simulink model "Master_Slave_Model"  (R2020b)
settings: Solver=VariableStepAuto  StartTime=0.0  StopTime=10  RelTol=1e-3
values from neighbouring files (symbols this model uses):
  A = [1 Ts;0 1]    [parameters_ACZC.m]
  Be = 5    [parameters_ACZC.m]
  beta = 2*pi*Fc*Ts / (1+2*pi*Fc*Ts)    (= 0.111635211705)    [parameters_ACZC.m]
  Bh = 2*0.7*sqrt(Kh)    [parameters_ACZC.m]
  C = [1 0]    [parameters_ACZC.m]
  delayCommM2S = 0    [parameters_ACZC.m]
  delayCommS2M = 0    [parameters_ACZC.m]
  dt = 0.001    [parameters_ACZC.m]
  Fc = 20    [parameters_ACZC.m]
  Jh = 0    [parameters_ACZC.m]
  k_m = 19.34    [parameters_ACZC.m]
  k_s = 19.34    [parameters_ACZC.m]
  Kc2v_m = 2    [parameters_ACZC.m]
  Kc2v_s = 2    [parameters_ACZC.m]
  Kd_h = 0.5    [parameters_ACZC.m]
  Kd_s = 1.5    [parameters_ACZC.m]
  Ke = 10    [parameters_ACZC.m]
  Kh = 2    [parameters_ACZC.m]
  Kh_max = 50    [parameters_ACZC.m]
  Kp_h = 1.2    [parameters_ACZC.m]
  Kp_s = 1    [parameters_ACZC.m]
  Kt2c_m = 1.182    [parameters_ACZC.m]
  Kt2c_s = 1.182    [parameters_ACZC.m]
  lArm_m = 0.1    [parameters_ACZC.m]
  lArm_s = 0.1    [parameters_ACZC.m]
  maxCurrent_m = 4.5    [parameters_ACZC.m]
  maxCurrent_s = 4.5    [parameters_ACZC.m]
  PosRef = 1    [parameters_ACZC.m]
  qe = 2    [parameters_ACZC.m]
  stopTime = str2double(stopTime)    [parameters_ACZC.m]
  tau_s = 1.217    [parameters_ACZC.m]
  Ts = 0.001    [parameters_ACZC.m]
  Variance = 0.0000001    (= 1e-07)    [parameters_ACZC.m]
undefined symbols (not defined in the file or in its folder): DiscIntNeverNeededParam, Discrete, Time
libraries: simulink_extras x20, dspsigops x20, ctrlSharedLib x7, cstblocks x1
settings Model: Creator=Mirko  LastModifiedBy=mirko

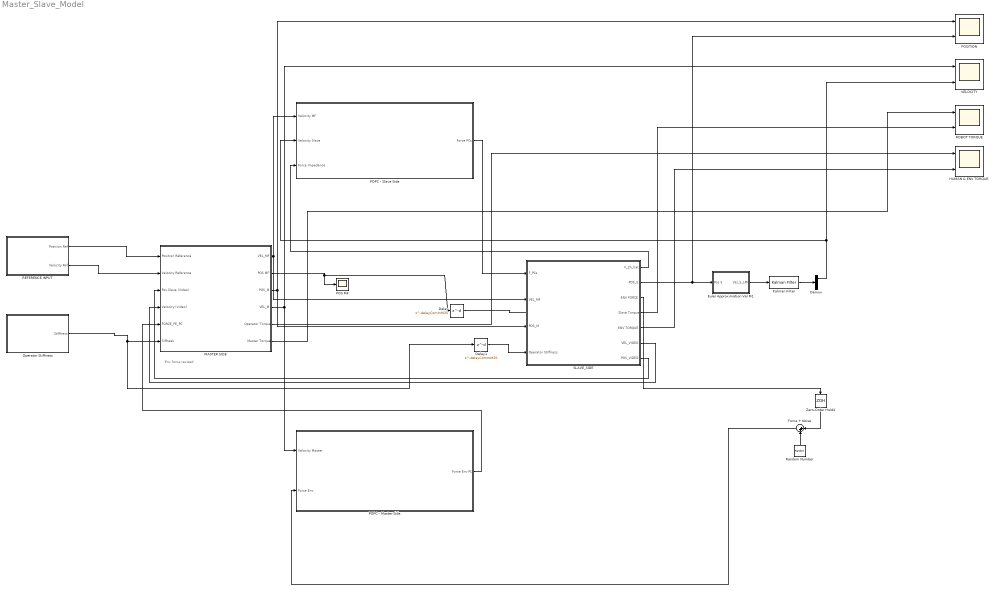
== system Master_Slave_Model ==
  note: Env force revised
  Delay : Delay  DelayLength=delayCommM2S  SampleTime=Ts
  Delay1 : Delay  DelayLength=delayCommM2S  SampleTime=Ts
  Demux : Demux  Outputs=2
  Euler Approximation Vel M1 : Subsystem
  Force + Noise : Sum  Inputs=|++
  HUMAN & ENV TORQUE : Scope  NumInputPorts=2
  Kalman Filter : ctrlSharedLib/Kalman Filter  TimeDomain=Discrete-Time  UseCurrentEstimator=off  ModelSource=Individual A, B, C, D matrices  ModelSourceVariable=ss(A,0,C,0)  A=A  B=1  C=C  D=0  NumberOfStates=2  NumberOfInputs=1  NumberOfOutputs=1  InitialEstimateSource=Dialog  X0=0  P0=10  UseK=off  UseGH=off  NumberOfProcessNoiseInputs=1  G=1  TimeInvariantG=on  H=0  TimeInvariantH=on  Q=0.05  TimeInvariantQ=on  R=1  TimeInvariantR=on  N=0  TimeInvariantN=on  AddInputPort=off  AddEnablePort=off  OutputEstimatedY=off  OutputP=off  Ts=Ts
  MASTER SIDE : Subsystem
  Operator Stiffness : Subsystem
  POPC - Master Side : Subsystem
  POPC - Slave Side : Subsystem
  "POS MF " : Scope
  "POSITION " : Scope  NumInputPorts=2
  REFERENCE INPUT : Subsystem
  ROBOT TORQUE : Scope  NumInputPorts=2
  Random Number : RandomNumber  Variance=Variance  SampleTime=Ts
  "SLAVE_SIDE " : Subsystem
  VELOCITY : Scope  NumInputPorts=2
  Zero-Order Hold4 : ZeroOrderHold  SampleTime=Ts
  wires:
  Delay1/1 -> "SLAVE_SIDE "/4(Operator Stiffness)
  Delay/1 -> ?
  Operator Stiffness/1(Stiffness) -> Delay1/1, MASTER SIDE/6(Siffness)
  "SLAVE_SIDE "/1(F_Zh_hat) -> POPC - Slave Side/3(Force Impedence)
  MASTER SIDE/2(POS MF) -> "POS MF "/1, Delay/1
  "SLAVE_SIDE "/2(POS_S) -> "POSITION "/2, Euler Approximation Vel M1/1(Pos S)
  MASTER SIDE/1(VEL_MF) -> "SLAVE_SIDE "/2(VEL_MF), POPC - Slave Side/1(Velocity MF)
  Demux/1 -> VELOCITY/2, POPC - Slave Side/2(Velocity Slave)
  Kalman Filter/1 -> Demux/1
  Euler Approximation Vel M1/1("Vel_S_LPF ") -> Kalman Filter/1
  POPC - Slave Side/1(Force PCs) -> "SLAVE_SIDE "/1(F_PCs)
  MASTER SIDE/4(VEL_M) -> POPC - Master Side/1(Velocity Master), VELOCITY/1
  Force + Noise/1 -> POPC - Master Side/2(Force Env)
  Zero-Order Hold4/1 -> Force + Noise/1
  Random Number/1 -> Force + Noise/2
  "SLAVE_SIDE "/3(ENV FORCE) -> Zero-Order Hold4/1
  POPC - Master Side/1(Force Env PC) -> MASTER SIDE/5("FORCE_FE_PC ")
  MASTER SIDE/3(POS_M) -> "SLAVE_SIDE "/3(POS_M), "POSITION "/1
  MASTER SIDE/5(Operator Torque) -> HUMAN & ENV TORQUE/1
  MASTER SIDE/6(Master Torque) -> ROBOT TORQUE/1
  REFERENCE INPUT/1("Position Ref ") -> MASTER SIDE/1(Position Reference)
  REFERENCE INPUT/2("Velocity Ref ") -> MASTER SIDE/2(Velocity Reference)
  "SLAVE_SIDE "/7(POS_VIDEO) -> MASTER SIDE/3(Pos Slave (Video))
  "SLAVE_SIDE "/6(VEL_VIDEO) -> MASTER SIDE/4(Velocity (Video))
  "SLAVE_SIDE "/4(Slave Torque) -> ROBOT TORQUE/2
  "SLAVE_SIDE "/5(ENV TORQUE) -> HUMAN & ENV TORQUE/2

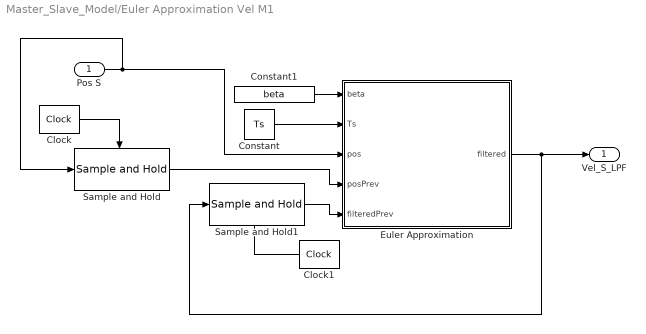
== system Master_Slave_Model/Euler Approximation Vel M1 ==
  Pos S : Inport
  Clock : simulink_extras/Flip Flops/Clock  period=Ts*2
  Clock1 : simulink_extras/Flip Flops/Clock  period=Ts*2
  Constant : Constant  Value=Ts
  Constant1 : Constant  Value=beta
  "Euler Approximation " : MATLAB Function  TreatAsAtomicUnit=on
  Sample and Hold : dspsigops/Sample and Hold  trig=Rising edge  initCond=0  latchinput=on
  Sample and Hold1 : dspsigops/Sample and Hold  trig=Rising edge  initCond=0  latchinput=on
  "Vel_S_LPF " : Outport
  wires:
  Pos S/1 -> Sample and Hold/1, "Euler Approximation "/3(pos)
  Constant/1 -> "Euler Approximation "/2(Ts)
  Sample and Hold/1 -> "Euler Approximation "/4(posPrev)
  Clock/1 -> Sample and Hold/Trigger
  Sample and Hold1/1 -> "Euler Approximation "/5(filteredPrev)
  "Euler Approximation "/1(filtered) -> "Vel_S_LPF "/1, Sample and Hold1/1
  Clock1/1 -> Sample and Hold1/Trigger
  Constant1/1 -> "Euler Approximation "/1(beta)

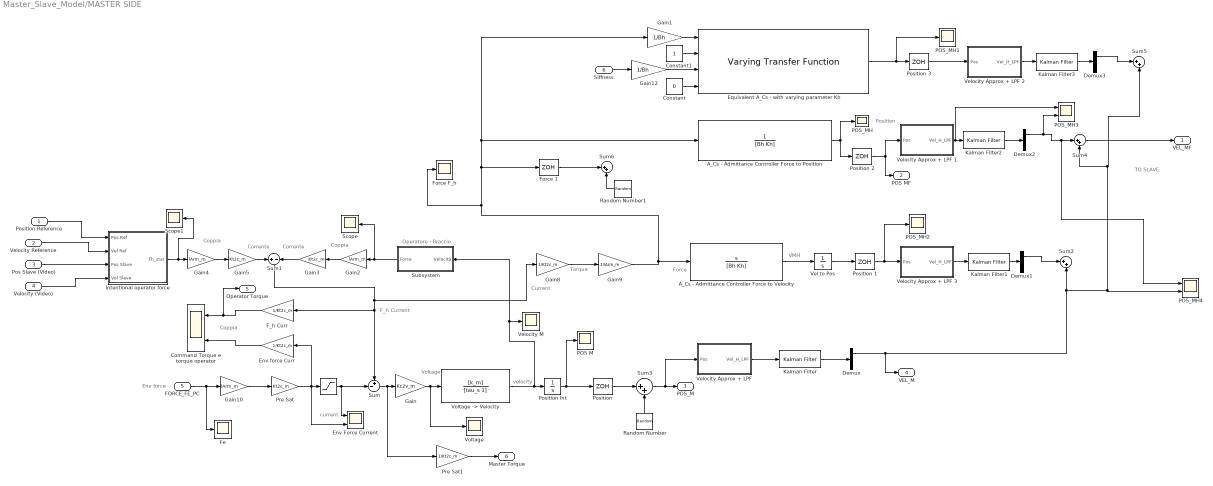
== system Master_Slave_Model/MASTER SIDE ==
  note: VMH
  note: Position
  note: Env force
  note: Force
  note: Torque
  note: Current
  note: F_h Current
  note: Coppia
  note: Corrente
  note: Coppia
  note: Corrente
  note: Coppia
  note: Operatore - Braccio
  note: current
  note: Voltage
  note: velocity
  note: TO SLAVE
  Position Reference : Inport
  Velocity Reference : Inport  Port=2
  Pos Slave (Video) : Inport  Port=3
  Velocity (Video) : Inport  Port=4
  "FORCE_FE_PC " : Inport  Port=5
  Siffness : Inport  Port=6
  " " : Saturate  UpperLimit=maxCurrent_m  LowerLimit=-maxCurrent_m
  A_Cs - Admittance Controller Force to Position : TransferFcn  Denominator=[Bh Kh]
  A_Cs - Admittance Controller Force to Velocity : TransferFcn  Numerator=[1 0]  Denominator=[Bh Kh]
  "Command Torque e torque operator " : Scope  NumInputPorts=2
  Constant : Constant  Value=0
  Constant1 : Constant
  Demux{,1..3} (4 alike) : Demux  Outputs=2
  Env Force Current : Scope  NumInputPorts=2
  Env force Curr : Gain  Gain=1/Kt2c_m
  Equivalent A_Cs - with varying parameter Kh : cstblocks/Linear Parameter Varying/Varying Transfer Function  N=1
  F_h Curr : Gain  Gain=1/Kt2c_m
  Fe : Scope
  Force 1 : ZeroOrderHold  SampleTime=Ts
  "Force F_h " : Scope
  Gain : Gain  Gain=Kc2v_m
  Gain1 : Gain  Gain=1/Bh
  Gain10 : Gain  Gain=lArm_m
  Gain12 : Gain  Gain=1/Bh
  Gain2 : Gain  Gain=lArm_m
  Gain3 : Gain  Gain=Kt2c_m
  Gain4 : Gain  Gain=lArm_m
  Gain5 : Gain  Gain=Kt2c_m
  Gain8 : Gain  Gain=1/Kt2c_m
  Gain9 : Gain  Gain=1/lArm_m
  Intentional operator force : Subsystem
  Kalman Filter{,1..3} (4 alike) : ctrlSharedLib/Kalman Filter  TimeDomain=Discrete-Time  UseCurrentEstimator=off  ModelSource=Individual A, B, C, D matrices  ModelSourceVariable=ss(A,0,C,0)  A=A  B=1  C=C  D=0  NumberOfStates=2  NumberOfInputs=1  NumberOfOutputs=1  InitialEstimateSource=Dialog  X0=0  P0=10  UseK=off  UseGH=off  NumberOfProcessNoiseInputs=1  G=1  TimeInvariantG=on  H=0  TimeInvariantH=on  Q=0.05  TimeInvariantQ=on  R=1  TimeInvariantR=on  N=0  TimeInvariantN=on  AddInputPort=off  AddEnablePort=off  OutputEstimatedY=off  OutputP=off  Ts=Ts
  "POS M " : Scope
  POS_MH : Scope
  POS_MH1 : Scope
  POS_MH2 : Scope
  POS_MH3 : Scope  NumInputPorts=2
  POS_MH4 : Scope  NumInputPorts=2
  Position {,1..3} (4 alike) : ZeroOrderHold  SampleTime=Ts
  "Position Int " : Integrator
  Pre Sat : Gain  Gain=Kt2c_m
  Pre Sat1 : Gain  Gain=1/Kt2c_m
  Random Number : RandomNumber  Variance=Variance  SampleTime=Ts
  Random Number1 : RandomNumber  Variance=Variance  SampleTime=0.1
  Scope : Scope
  Scope1 : Scope
  Subsystem : Subsystem
  Sum : Sum  Inputs=+-|
  Sum1 : Sum  Inputs=+-
  Sum{2..6} (5 alike) : Sum  Inputs=|++
  Vel to Pos : Integrator
  "Velocity Approx + LPF " : Subsystem
  Velocity Approx + LPF 1 : Subsystem
  Velocity Approx + LPF 2 : Subsystem
  Velocity Approx + LPF 3 : Subsystem
  Velocity M : Scope
  Voltage : Scope
  "Voltage -> Velocity" : TransferFcn  Numerator=[k_m]  Denominator=[tau_s 1]
  VEL_MF : Outport
  POS MF : Outport  Port=2
  POS_M : Outport  Port=3
  VEL_M : Outport  Port=4
  Operator Torque : Outport  Port=5
  Master Torque : Outport  Port=6
  wires:
  Pre Sat/1 -> Env Force Current/2, Env force Curr/1, " "/1
  "Position Int "/1 -> "Position "/1, "POS M "/1
  "Voltage -> Velocity"/1 -> Velocity M/1, Subsystem/1("Velocità "), "Position Int "/1
  Sum1/1 -> Sum/1, F_h Curr/1, Gain8/1
  Gain4/1 -> Gain5/1
  F_h Curr/1 -> Operator Torque/1, "Command Torque e torque operator "/1
  Gain2/1 -> Gain3/1
  Gain3/1 -> Sum1/2
  Env force Curr/1 -> "Command Torque e torque operator "/2
  Gain5/1 -> Sum1/1
  Gain/1 -> "Voltage -> Velocity"/1, Voltage/1
  Velocity Approx + LPF 3/1("Vel_H_LPF ") -> Kalman Filter1/1
  Gain8/1 -> Gain9/1
  Gain9/1 -> Force 1/1, Gain1/1, A_Cs - Admittance Controller Force to Position/1, "Force F_h "/1, A_Cs - Admittance Controller Force to Velocity/1
  "FORCE_FE_PC "/1 -> Fe/1, Gain10/1
  Gain10/1 -> Pre Sat/1
  Constant/1 -> Equivalent A_Cs - with varying parameter Kh/4
  Gain12/1 -> Equivalent A_Cs - with varying parameter Kh/3
  Siffness/1 -> Gain12/1
  Constant1/1 -> Equivalent A_Cs - with varying parameter Kh/2
  Equivalent A_Cs - with varying parameter Kh/1 -> Position 3/1, POS_MH1/1
  Subsystem/1(Force) -> Scope/1, Gain2/1
  A_Cs - Admittance Controller Force to Position/1 -> Position 2/1, POS_MH/1
  Sum4/1 -> VEL_MF/1
  Gain1/1 -> Equivalent A_Cs - with varying parameter Kh/1
  Velocity Approx + LPF 1/1("Vel_H_LPF ") -> POS_MH3/1, Kalman Filter2/1
  Velocity Approx + LPF 2/1("Vel_H_LPF ") -> Kalman Filter3/1
  " "/1 -> Sum/2, Env Force Current/1
  Random Number/1 -> Sum3/2
  Sum3/1 -> "Velocity Approx + LPF "/1(Pos), POS_M/1
  "Velocity Approx + LPF "/1("Vel_H_LPF ") -> Kalman Filter/1
  "Position "/1 -> Sum3/1
  Velocity (Video)/1 -> Intentional operator force/4(Vel Slave)
  Pos Slave (Video)/1 -> Intentional operator force/3(Pos Slave)
  Position Reference/1 -> Intentional operator force/1(Pos Ref)
  Velocity Reference/1 -> Intentional operator force/2(Vel Ref)
  Intentional operator force/1("Fh_star ") -> Scope1/1, Gain4/1
  Random Number1/1 -> Sum6/2
  Force 1/1 -> Sum6/1
  Demux/1 -> Sum2/2, Sum4/2, Sum5/2, POS_MH4/2, VEL_M/1
  Kalman Filter/1 -> Demux/1
  A_Cs - Admittance Controller Force to Velocity/1 -> Vel to Pos/1
  Position 1/1 -> Velocity Approx + LPF 3/1(Pos), POS_MH2/1
  Demux1/1 -> Sum2/1
  Kalman Filter1/1 -> Demux1/1
  Demux2/1 -> POS_MH3/2, POS_MH4/1, Sum4/1
  Kalman Filter2/1 -> Demux2/1
  Vel to Pos/1 -> Position 1/1
  Position 2/1 -> Velocity Approx + LPF 1/1(Pos), POS MF/1
  Position 3/1 -> Velocity Approx + LPF 2/1(Pos)
  Demux3/1 -> Sum5/1
  Kalman Filter3/1 -> Demux3/1
  Pre Sat1/1 -> Master Torque/1
  Sum/1 -> Pre Sat1/1, Gain/1

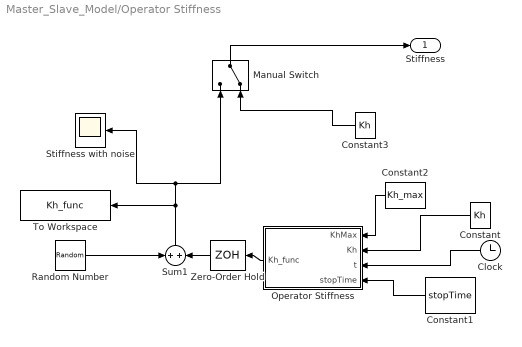
== system Master_Slave_Model/Operator Stiffness ==
  Clock : Clock
  Constant : Constant  Value=Kh
  Constant1 : Constant  Value=stopTime  SampleTime=Ts
  Constant2 : Constant  Value=Kh_max
  Constant3 : Constant  Value=Kh
  Manual Switch : ManualSwitch  CurrentSetting=0
  "Operator Stiffness " : MATLAB Function  TreatAsAtomicUnit=on
  Random Number : RandomNumber  Variance=Variance  SampleTime=Ts
  Stiffness with noise : Scope
  Sum1 : Sum
  To Workspace : ToWorkspace  VariableName=Kh_func  SaveFormat=Structure With Time  SampleTime=-1
      settings: Save2DSignal=2-D array (concatenate along first dimension)
  Zero-Order Hold : ZeroOrderHold  SampleTime=-1
  Stiffness : Outport
  wires:
  Constant3/1 -> Manual Switch/2
  Sum1/1 -> To Workspace/1, Manual Switch/1, Stiffness with noise/1
  Constant2/1 -> "Operator Stiffness "/1(KhMax)
  "Operator Stiffness "/1(Kh_func) -> Zero-Order Hold/1
  Clock/1 -> "Operator Stiffness "/3(t)
  Random Number/1 -> Sum1/1
  Constant/1 -> "Operator Stiffness "/2(Kh)
  Constant1/1 -> "Operator Stiffness "/4(stopTime)
  Manual Switch/1 -> Stiffness/1
  Zero-Order Hold/1 -> Sum1/2

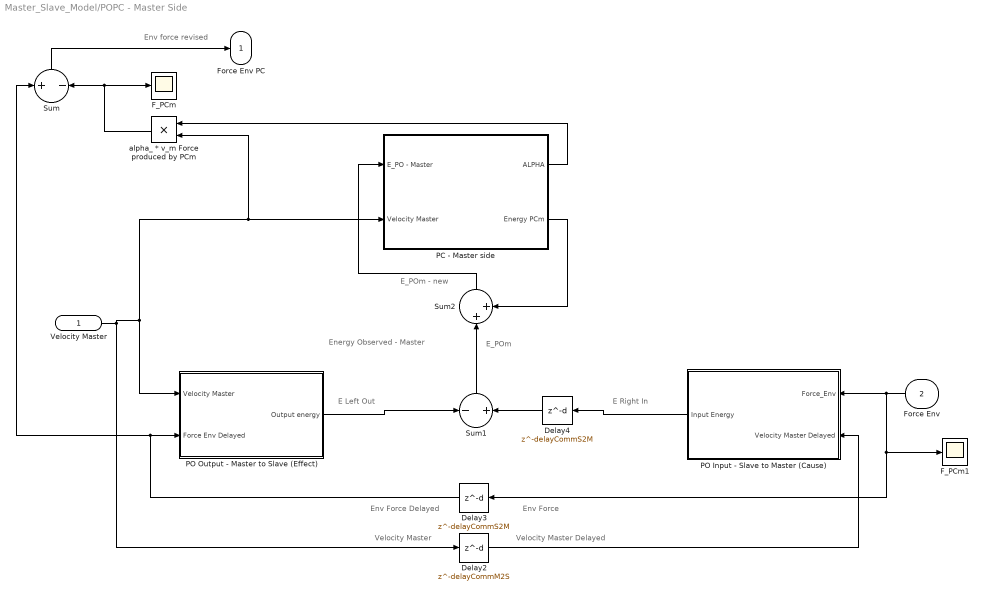
== system Master_Slave_Model/POPC - Master Side ==
  note: E_POm
  note: Energy Observed - Master
  note: Env force revised
  note: Env Force Delayed
  note: Env Force
  note: Velocity Master
  note: Velocity Master Delayed
  note: E Left Out
  note: E Right In
  note: E_POm - new
  Velocity Master : Inport
  Force Env : Inport  Port=2
  Delay2 : Delay  DelayLength=delayCommM2S  InitialCondition=0  SampleTime=Ts
  Delay3 : Delay  DelayLength=delayCommS2M  InitialCondition=0  SampleTime=Ts
  Delay4 : Delay  DelayLength=delayCommS2M  InitialCondition=0
  F_PCm : Scope
  F_PCm1 : Scope
  PC - Master side : Subsystem
  PO Input - Slave to Master (Cause) : Subsystem
  PO Output - Master to Slave (Effect) : Subsystem
  Sum : Sum  Inputs=+-
  Sum1 : Sum  Inputs=-+
  Sum2 : Sum  Inputs=|++
  alpha_ * v_m Force produced by PCm : Product
  Force Env PC : Outport
  wires:
  alpha_ * v_m Force produced by PCm/1 -> Sum/2, F_PCm/1
  Force Env/1 -> Delay3/1, F_PCm1/1, PO Input - Slave to Master (Cause)/1(Force_Env)
  Delay3/1 -> Sum/1, PO Output - Master to Slave (Effect)/2(Force Env Delayed)
  Velocity Master/1 -> Delay2/1, alpha_ * v_m Force produced by PCm/2, PC - Master side/2("Velocity Master "), PO Output - Master to Slave (Effect)/1(Velocity Master)
  Sum1/1 -> Sum2/1
  Sum/1 -> Force Env PC/1
  PO Output - Master to Slave (Effect)/1(Output energy) -> Sum1/1
  Delay4/1 -> Sum1/2
  Delay2/1 -> PO Input - Slave to Master (Cause)/2(Velocity Master Delayed)
  PO Input - Slave to Master (Cause)/1(Input Energy) -> Delay4/1
  Sum2/1 -> PC - Master side/1(E_PO - Master)
  PC - Master side/1(ALPHA) -> alpha_ * v_m Force produced by PCm/1
  PC - Master side/2(Energy PCm) -> Sum2/2

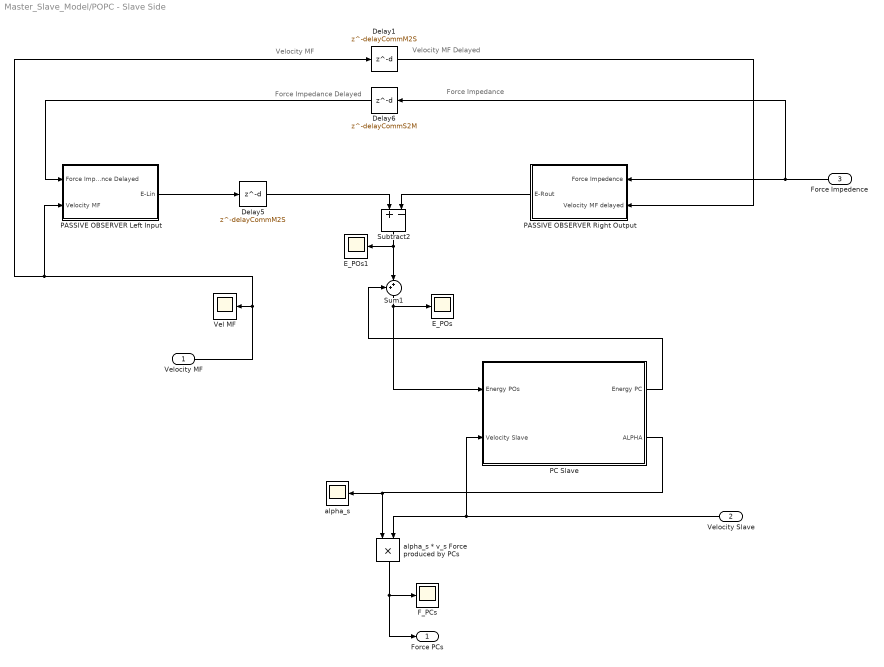
== system Master_Slave_Model/POPC - Slave Side ==
  note: Velocity MF Delayed
  note: Velocity MF
  note: Force Impedance Delayed
  note: Force Impedance
  Velocity MF : Inport
  Velocity Slave : Inport  Port=2
  Force Impedence : Inport  Port=3
  Delay1 : Delay  DelayLength=delayCommM2S  InitialCondition=0  SampleTime=Ts
  Delay5 : Delay  DelayLength=delayCommM2S  InitialCondition=0  SampleTime=Ts
  Delay6 : Delay  DelayLength=delayCommS2M  InitialCondition=0  SampleTime=Ts
  E_POs : Scope
  E_POs1 : Scope
  F_PCs : Scope
  PASSIVE OBSERVER Left Input : Subsystem
  PASSIVE OBSERVER Right Output : Subsystem
  PC Slave : Subsystem
  Subtract2 : Sum  Inputs=+|-
  Sum1 : Sum  Inputs=++|
  Vel MF : Scope
  alpha_s : Scope
  alpha_s * v_s Force produced by PCs : Product
  Force PCs : Outport
  wires:
  Subtract2/1 -> E_POs1/1, Sum1/2
  Delay6/1 -> PASSIVE OBSERVER Left Input/1(Force Impedance Delayed)
  Velocity Slave/1 -> alpha_s * v_s Force produced by PCs/2, PC Slave/2(Velocity Slave)
  Sum1/1 -> PC Slave/1(Energy POs), E_POs/1
  Delay5/1 -> Subtract2/1
  alpha_s * v_s Force produced by PCs/1 -> Force PCs/1, F_PCs/1
  PASSIVE OBSERVER Left Input/1(E-Lin) -> Delay5/1
  Velocity MF/1 -> PASSIVE OBSERVER Left Input/2(Velocity MF), Delay1/1, Vel MF/1
  PASSIVE OBSERVER Right Output/1(E-Rout) -> Subtract2/2
  Force Impedence/1 -> Delay6/1, PASSIVE OBSERVER Right Output/1(Force Impedence)
  Delay1/1 -> PASSIVE OBSERVER Right Output/2(Velocity MF delayed)
  PC Slave/2(ALPHA) -> alpha_s * v_s Force produced by PCs/1, alpha_s/1
  PC Slave/1(Energy PC) -> Sum1/1

== system Master_Slave_Model/REFERENCE INPUT ==
  Derivative : Derivative
  Manual Switch : ManualSwitch  CurrentSetting=0
  Scope : Scope
  Sine Wave : Sin  Amplitude=PosRef  SampleTime=0
  Step : Step  After=PosRef  SampleTime=0
  Transfer Fcn : TransferFcn  Numerator=[2*pi*Fc]  Denominator=[1 2*pi*Fc]
  "Position Ref " : Outport
  "Velocity Ref " : Outport  Port=2
  wires:
  Sine Wave/1 -> Manual Switch/1
  Derivative/1 -> "Velocity Ref "/1
  Manual Switch/1 -> Derivative/1, "Position Ref "/1
  Transfer Fcn/1 -> Scope/1, Manual Switch/2
  Step/1 -> Transfer Fcn/1

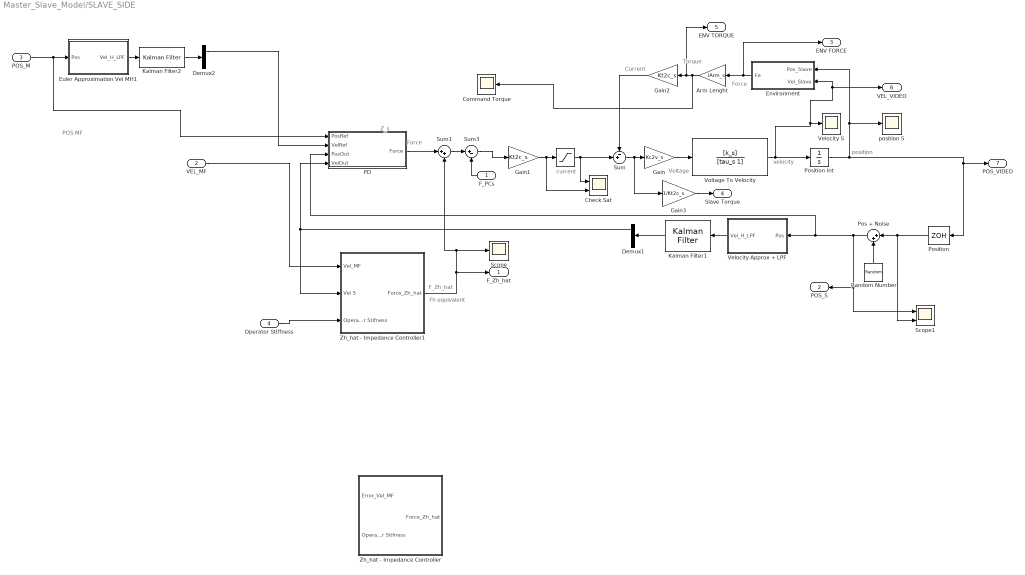
== system Master_Slave_Model/SLAVE_SIDE  ==
  note: Fh equivalent
  note: POS MF
  note: current
  note: Force
  note: velocity
  note: position
  note: Current
  note: Voltage
  note: Torque
  note: Z_s
  note: Force
  note: F_Zh_hat
  F_PCs : Inport
  VEL_MF : Inport  Port=2
  POS_M : Inport  Port=3
  Operator Stiffness : Inport  Port=4
  " " : Saturate  UpperLimit=maxCurrent_s  LowerLimit=-maxCurrent_s
  Arm Lenght : Gain  Gain=lArm_s
  Check Sat : Scope  NumInputPorts=2
  Command Torque : Scope
  Demux1 : Demux  Outputs=2
  Demux2 : Demux  Outputs=2
  "Environment " : Subsystem
  Euler Approximation Vel MH1 : Subsystem
  Gain : Gain  Gain=Kc2v_s
  Gain1 : Gain  Gain=Kt2c_s
  Gain2 : Gain  Gain=Kt2c_s
  Gain3 : Gain  Gain=1/Kt2c_s
  Kalman Filter1 : ctrlSharedLib/Kalman Filter  TimeDomain=Discrete-Time  UseCurrentEstimator=off  ModelSource=Individual A, B, C, D matrices  ModelSourceVariable=ss(A,0,C,0)  A=A  B=1  C=C  D=0  NumberOfStates=2  NumberOfInputs=1  NumberOfOutputs=1  InitialEstimateSource=Dialog  X0=0  P0=10  UseK=off  UseGH=off  NumberOfProcessNoiseInputs=1  G=1  TimeInvariantG=on  H=0  TimeInvariantH=on  Q=0.05  TimeInvariantQ=on  R=1  TimeInvariantR=on  N=0  TimeInvariantN=on  AddInputPort=off  AddEnablePort=off  OutputEstimatedY=off  OutputP=off  Ts=Ts
  Kalman Filter2 : ctrlSharedLib/Kalman Filter  TimeDomain=Discrete-Time  UseCurrentEstimator=off  ModelSource=Individual A, B, C, D matrices  ModelSourceVariable=ss(A,0,C,0)  A=A  B=1  C=C  D=0  NumberOfStates=2  NumberOfInputs=1  NumberOfOutputs=1  InitialEstimateSource=Dialog  X0=0  P0=10  UseK=off  UseGH=off  NumberOfProcessNoiseInputs=1  G=1  TimeInvariantG=on  H=0  TimeInvariantH=on  Q=0.05  TimeInvariantQ=on  R=1  TimeInvariantR=on  N=0  TimeInvariantN=on  AddInputPort=off  AddEnablePort=off  OutputEstimatedY=off  OutputP=off  Ts=Ts
  PD : Subsystem
  Pos + Noise : Sum  Inputs=|++
  Position : ZeroOrderHold  SampleTime=Ts
  "Position Int " : Integrator
  Random Number : RandomNumber  Variance=Variance  SampleTime=Ts
  Scope : Scope
  Scope1 : Scope  NumInputPorts=2
  Sum : Sum  Inputs=-+|
  Sum1 : Sum  Inputs=|++
  Sum3 : Sum  Inputs=|+-
  "Velocity Approx + LPF " : Subsystem
  Velocity S : Scope
  "Voltage To Velocity " : TransferFcn  Numerator=[k_s]  Denominator=[tau_s 1]
  Zh_hat - Impedance Controller : Subsystem
  Zh_hat - Impedance Controller1 : Subsystem
  "position S " : Scope
  F_Zh_hat : Outport
  POS_S : Outport  Port=2
  ENV FORCE : Outport  Port=3
  Slave Torque : Outport  Port=4
  ENV TORQUE : Outport  Port=5
  VEL_VIDEO : Outport  Port=6
  POS_VIDEO : Outport  Port=7
  wires:
  PD/1(Force) -> Sum1/1
  "Position Int "/1 -> Position/1, POS_VIDEO/1, "position S "/1, "Environment "/1(Pos_Slave)
  Gain1/1 -> Check Sat/2, " "/1
  Gain2/1 -> Sum/1
  "Environment "/1(Fe) -> ENV FORCE/1, Arm Lenght/1
  "Voltage To Velocity "/1 -> "Position Int "/1, Velocity S/1, "Environment "/2("Vel_Slave "), VEL_VIDEO/1
  Sum/1 -> Gain3/1, Gain/1
  Gain/1 -> "Voltage To Velocity "/1
  Sum1/1 -> Sum3/1
  " "/1 -> Check Sat/1, Sum/2
  Arm Lenght/1 -> Command Torque/1, ENV TORQUE/1, Gain2/1
  Zh_hat - Impedance Controller1/1("Force_Zh_hat ") -> Sum1/2, Scope/1, F_Zh_hat/1
  F_PCs/1 -> Sum3/2
  Operator Stiffness/1 -> Zh_hat - Impedance Controller1/3(Operator Stifness)
  VEL_MF/1 -> Zh_hat - Impedance Controller1/1(Vel_MF)
  Pos + Noise/1 -> PD/3(PosOut), "Velocity Approx + LPF "/1(Pos), POS_S/1, Scope1/1
  Random Number/1 -> Pos + Noise/2
  Demux1/1 -> PD/4(VelOut), Zh_hat - Impedance Controller1/2(Vel S)
  Position/1 -> Scope1/2, Pos + Noise/1
  "Velocity Approx + LPF "/1("Vel_H_LPF ") -> Kalman Filter1/1
  Kalman Filter1/1 -> Demux1/1
  Gain3/1 -> Slave Torque/1
  POS_M/1 -> PD/1(PosRef), Euler Approximation Vel MH1/1(Pos)
  Euler Approximation Vel MH1/1("Vel_H_LPF ") -> Kalman Filter2/1
  Kalman Filter2/1 -> Demux2/1
  Demux2/1 -> PD/2(VelRef)
  Sum3/1 -> Gain1/1

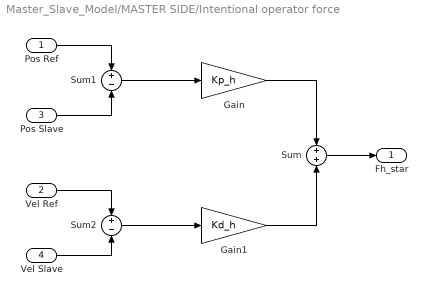
== system Master_Slave_Model/MASTER SIDE/Intentional operator force ==
  Pos Ref : Inport
  Vel Ref : Inport  Port=2
  Pos Slave : Inport  Port=3
  Vel Slave : Inport  Port=4
  Gain : Gain  Gain=Kp_h
  Gain1 : Gain  Gain=Kd_h
  Sum : Sum
  Sum1 : Sum  Inputs=+-
  Sum2 : Sum  Inputs=+-
  "Fh_star " : Outport
  wires:
  Sum/1 -> "Fh_star "/1
  Pos Ref/1 -> Sum1/1
  Pos Slave/1 -> Sum1/2
  Vel Ref/1 -> Sum2/1
  Vel Slave/1 -> Sum2/2
  Sum1/1 -> Gain/1
  Sum2/1 -> Gain1/1
  Gain1/1 -> Sum/2
  Gain/1 -> Sum/1

== system Master_Slave_Model/MASTER SIDE/Subsystem ==
  "Velocità " : Inport
  Derivative : Derivative  CoefficientInTFapproximation=0.01
  Friction : Gain  Gain=Bh
  Inertia : Gain  Gain=Jh
  Integrator : Integrator
  "Stiffness " : Gain  Gain=Kh
  Sum : Sum  Inputs=+++
  Force : Outport
  wires:
  "Velocità "/1 -> Friction/1, Integrator/1, Derivative/1
  Derivative/1 -> Inertia/1
  Inertia/1 -> Sum/2
  Friction/1 -> Sum/1
  Sum/1 -> Force/1
  Integrator/1 -> "Stiffness "/1
  "Stiffness "/1 -> Sum/3

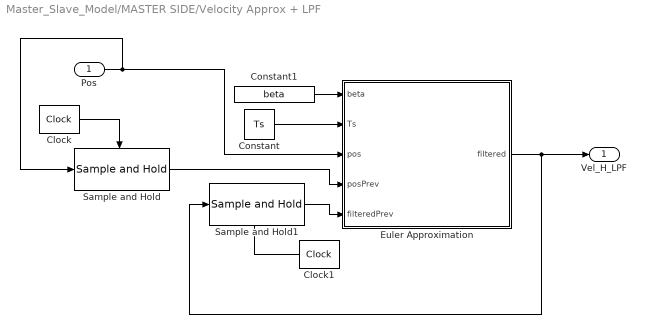
== system Master_Slave_Model/MASTER SIDE/Velocity Approx + LPF  ==
  Pos : Inport
  Clock : simulink_extras/Flip Flops/Clock  period=Ts*2
  Clock1 : simulink_extras/Flip Flops/Clock  period=Ts*2
  Constant : Constant  Value=Ts
  Constant1 : Constant  Value=beta
  "Euler Approximation " : MATLAB Function  TreatAsAtomicUnit=on
  Sample and Hold : dspsigops/Sample and Hold  trig=Rising edge  initCond=0  latchinput=on
  Sample and Hold1 : dspsigops/Sample and Hold  trig=Rising edge  initCond=0  latchinput=on
  "Vel_H_LPF " : Outport
  wires:
  Pos/1 -> Sample and Hold/1, "Euler Approximation "/3(pos)
  Constant/1 -> "Euler Approximation "/2(Ts)
  Sample and Hold/1 -> "Euler Approximation "/4(posPrev)
  Clock/1 -> Sample and Hold/Trigger
  Sample and Hold1/1 -> "Euler Approximation "/5(filteredPrev)
  "Euler Approximation "/1(filtered) -> "Vel_H_LPF "/1, Sample and Hold1/1
  Clock1/1 -> Sample and Hold1/Trigger
  Constant1/1 -> "Euler Approximation "/1(beta)

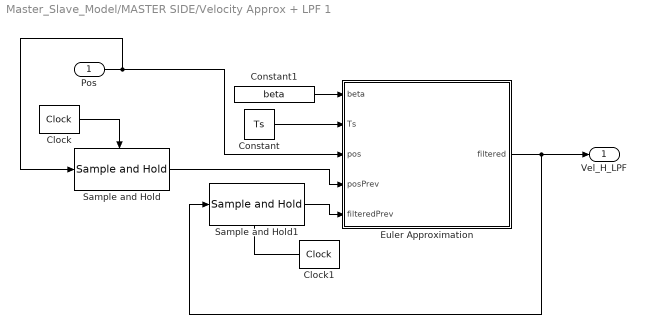
== system Master_Slave_Model/MASTER SIDE/Velocity Approx + LPF 1 ==
  Pos : Inport
  Clock : simulink_extras/Flip Flops/Clock  period=Ts*2
  Clock1 : simulink_extras/Flip Flops/Clock  period=Ts*2
  Constant : Constant  Value=Ts
  Constant1 : Constant  Value=beta
  "Euler Approximation " : MATLAB Function  TreatAsAtomicUnit=on
  Sample and Hold : dspsigops/Sample and Hold  trig=Rising edge  initCond=0  latchinput=on
  Sample and Hold1 : dspsigops/Sample and Hold  trig=Rising edge  initCond=0  latchinput=on
  "Vel_H_LPF " : Outport
  wires:
  Pos/1 -> Sample and Hold/1, "Euler Approximation "/3(pos)
  Constant/1 -> "Euler Approximation "/2(Ts)
  Sample and Hold/1 -> "Euler Approximation "/4(posPrev)
  Clock/1 -> Sample and Hold/Trigger
  Sample and Hold1/1 -> "Euler Approximation "/5(filteredPrev)
  "Euler Approximation "/1(filtered) -> "Vel_H_LPF "/1, Sample and Hold1/1
  Clock1/1 -> Sample and Hold1/Trigger
  Constant1/1 -> "Euler Approximation "/1(beta)

== system Master_Slave_Model/MASTER SIDE/Velocity Approx + LPF 2 ==
  Pos : Inport
  Clock : simulink_extras/Flip Flops/Clock  period=Ts*2
  Clock1 : simulink_extras/Flip Flops/Clock  period=Ts*2
  Constant : Constant  Value=Ts
  Constant1 : Constant  Value=beta
  "Euler Approximation " : MATLAB Function  TreatAsAtomicUnit=on
  Sample and Hold : dspsigops/Sample and Hold  trig=Rising edge  initCond=0  latchinput=on
  Sample and Hold1 : dspsigops/Sample and Hold  trig=Rising edge  initCond=0  latchinput=on
  "Vel_H_LPF " : Outport
  wires:
  Pos/1 -> Sample and Hold/1, "Euler Approximation "/3(pos)
  Constant/1 -> "Euler Approximation "/2(Ts)
  Sample and Hold/1 -> "Euler Approximation "/4(posPrev)
  Clock/1 -> Sample and Hold/Trigger
  Sample and Hold1/1 -> "Euler Approximation "/5(filteredPrev)
  "Euler Approximation "/1(filtered) -> "Vel_H_LPF "/1, Sample and Hold1/1
  Clock1/1 -> Sample and Hold1/Trigger
  Constant1/1 -> "Euler Approximation "/1(beta)

== system Master_Slave_Model/MASTER SIDE/Velocity Approx + LPF 3 ==
  Pos : Inport
  Clock : simulink_extras/Flip Flops/Clock  period=Ts*2
  Clock1 : simulink_extras/Flip Flops/Clock  period=Ts*2
  Constant : Constant  Value=Ts
  Constant1 : Constant  Value=beta
  "Euler Approximation " : MATLAB Function  TreatAsAtomicUnit=on
  Sample and Hold : dspsigops/Sample and Hold  trig=Rising edge  initCond=0  latchinput=on
  Sample and Hold1 : dspsigops/Sample and Hold  trig=Rising edge  initCond=0  latchinput=on
  "Vel_H_LPF " : Outport
  wires:
  Pos/1 -> Sample and Hold/1, "Euler Approximation "/3(pos)
  Constant/1 -> "Euler Approximation "/2(Ts)
  Sample and Hold/1 -> "Euler Approximation "/4(posPrev)
  Clock/1 -> Sample and Hold/Trigger
  Sample and Hold1/1 -> "Euler Approximation "/5(filteredPrev)
  "Euler Approximation "/1(filtered) -> "Vel_H_LPF "/1, Sample and Hold1/1
  Clock1/1 -> Sample and Hold1/Trigger
  Constant1/1 -> "Euler Approximation "/1(beta)

== system Master_Slave_Model/POPC - Master Side/PC - Master side ==
  E_PO - Master : Inport
  "Velocity Master " : Inport  Port=2
  Clock : simulink_extras/Flip Flops/Clock  period=Ts*2
  E_POm : Scope
  PASSIVE CONTROLLER PCm : MATLAB Function  TreatAsAtomicUnit=on
  Sample and Hold : dspsigops/Sample and Hold  trig=Rising edge  initCond=0  latchinput=on
  dt : Constant  Value=Ts
  ALPHA : Outport
  Energy PCm : Outport  Port=2
  wires:
  Sample and Hold/1 -> PASSIVE CONTROLLER PCm/4(E_PCm_prev)
  dt/1 -> PASSIVE CONTROLLER PCm/2(dt)
  E_PO - Master/1 -> E_POm/1, PASSIVE CONTROLLER PCm/1(E_POm)
  Clock/1 -> Sample and Hold/Trigger
  PASSIVE CONTROLLER PCm/1(E_PCm) -> Sample and Hold/1, Energy PCm/1
  PASSIVE CONTROLLER PCm/2(alpha_m) -> ALPHA/1
  "Velocity Master "/1 -> PASSIVE CONTROLLER PCm/3(v_m)

== system Master_Slave_Model/POPC - Master Side/PO Input - Slave to Master (Cause) ==
  Force_Env : Inport
  Velocity Master Delayed : Inport  Port=2
  E_Rin : Scope
  PASSIVE OBSERVER S2M E Right INPUT : Subsystem
  Input Energy : Outport
  wires:
  PASSIVE OBSERVER S2M E Right INPUT/1(E-Rin) -> Input Energy/1, E_Rin/1
  Velocity Master Delayed/1 -> PASSIVE OBSERVER S2M E Right INPUT/2("Vel_M ")
  Force_Env/1 -> PASSIVE OBSERVER S2M E Right INPUT/1(Env_Force)

== system Master_Slave_Model/POPC - Master Side/PO Output - Master to Slave (Effect) ==
  note: E Left Out
  Velocity Master : Inport
  Force Env Delayed : Inport  Port=2
  E_Lout : Scope
  PASSIVE OBSERVER M2S E Left OUTPUT : Subsystem
  Output energy : Outport
  wires:
  Velocity Master/1 -> PASSIVE OBSERVER M2S E Left OUTPUT/1(Velocity Master)
  PASSIVE OBSERVER M2S E Left OUTPUT/1(E-Lout) -> Output energy/1, E_Lout/1
  Force Env Delayed/1 -> PASSIVE OBSERVER M2S E Left OUTPUT/2(Force Env Delayed)

== system Master_Slave_Model/POPC - Slave Side/PASSIVE OBSERVER Left Input ==
  Force Impedance Delayed : Inport
  Velocity MF : Inport  Port=2
  Add : Sum
  Clock : simulink_extras/Flip Flops/Clock  period=Ts*2
  Product : Product
  Sample and Hold : dspsigops/Sample and Hold  trig=Rising edge  initCond=0  latchinput=on
  E-Lin : Outport
  wires:
  Velocity MF/1 -> Product/1
  Force Impedance Delayed/1 -> Product/2
  Product/1 -> Add/2
  Sample and Hold/1 -> Add/1
  Add/1 -> Sample and Hold/1, E-Lin/1
  Clock/1 -> Sample and Hold/Trigger

== system Master_Slave_Model/POPC - Slave Side/PASSIVE OBSERVER Right Output ==
  Force Impedence : Inport
  Velocity MF delayed : Inport  Port=2
  Add : Sum
  Clock : simulink_extras/Flip Flops/Clock  period=Ts*2
  Product : Product
  Sample and Hold : dspsigops/Sample and Hold  trig=Rising edge  initCond=0  latchinput=on
  E-Rout : Outport
  wires:
  Velocity MF delayed/1 -> Product/1
  Force Impedence/1 -> Product/2
  Product/1 -> Add/2
  Sample and Hold/1 -> Add/1
  Add/1 -> Sample and Hold/1, E-Rout/1
  Clock/1 -> Sample and Hold/Trigger

== system Master_Slave_Model/POPC - Slave Side/PC Slave ==
  Energy POs : Inport
  Velocity Slave : Inport  Port=2
  Clock1 : simulink_extras/Flip Flops/Clock  period=Ts*2
  PASSIVE CONTROLLER PCs : MATLAB Function  TreatAsAtomicUnit=on
  Sample and Hold1 : dspsigops/Sample and Hold  trig=Rising edge  initCond=0  latchinput=on
  dt1 : Constant  Value=dt
  Energy PC : Outport
  ALPHA : Outport  Port=2
  wires:
  PASSIVE CONTROLLER PCs/1(E_PCs) -> Sample and Hold1/1
  dt1/1 -> PASSIVE CONTROLLER PCs/3(dt)
  PASSIVE CONTROLLER PCs/2(alpha_s) -> ALPHA/1
  Energy POs/1 -> PASSIVE CONTROLLER PCs/2(E_POs)
  Clock1/1 -> Sample and Hold1/Trigger
  Sample and Hold1/1 -> Energy PC/1, PASSIVE CONTROLLER PCs/1(E_PCs_prev)
  Velocity Slave/1 -> PASSIVE CONTROLLER PCs/4(v_s)

== system Master_Slave_Model/SLAVE_SIDE /Environment  ==
  Pos_Slave : Inport
  "Vel_Slave " : Inport  Port=2
  Environment Behaviour : MATLAB Function  TreatAsAtomicUnit=on
  Environment Position : Constant  Value=qe
  Stiffness : Constant  Value=Ke
  Viscous Friction : Constant  Value=Be
  Fe : Outport
  wires:
  Pos_Slave/1 -> Environment Behaviour/1(x_s)
  "Vel_Slave "/1 -> Environment Behaviour/2(dot_x_s)
  Environment Position/1 -> Environment Behaviour/3(qe)
  Viscous Friction/1 -> Environment Behaviour/4(Be)
  Stiffness/1 -> Environment Behaviour/5(Ke)
  Environment Behaviour/1(Fe) -> Fe/1

== system Master_Slave_Model/SLAVE_SIDE /Euler Approximation Vel MH1 ==
  Pos : Inport
  Clock : simulink_extras/Flip Flops/Clock  period=Ts*2
  Clock1 : simulink_extras/Flip Flops/Clock  period=Ts*2
  Constant : Constant  Value=Ts
  Constant1 : Constant  Value=beta
  "Euler Approximation " : MATLAB Function  TreatAsAtomicUnit=on
  Sample and Hold : dspsigops/Sample and Hold  trig=Rising edge  initCond=0  latchinput=on
  Sample and Hold1 : dspsigops/Sample and Hold  trig=Rising edge  initCond=0  latchinput=on
  "Vel_H_LPF " : Outport
  wires:
  Constant1/1 -> "Euler Approximation "/1(beta)
  Clock1/1 -> Sample and Hold1/Trigger
  "Euler Approximation "/1(filtered) -> Sample and Hold1/1, "Vel_H_LPF "/1
  Sample and Hold1/1 -> "Euler Approximation "/5(filteredPrev)
  Clock/1 -> Sample and Hold/Trigger
  Sample and Hold/1 -> "Euler Approximation "/4(posPrev)
  Constant/1 -> "Euler Approximation "/2(Ts)
  Pos/1 -> "Euler Approximation "/3(pos), Sample and Hold/1

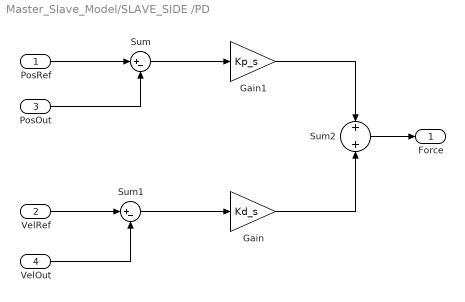
== system Master_Slave_Model/SLAVE_SIDE /PD ==
  PosRef : Inport
  VelRef : Inport  Port=2
  PosOut : Inport  Port=3
  VelOut : Inport  Port=4
  Gain : Gain  Gain=Kd_s
  Gain1 : Gain  Gain=Kp_s
  Sum : Sum  Inputs=|+-
  Sum1 : Sum  Inputs=|+-
  Sum2 : Sum
  Force : Outport
  wires:
  PosRef/1 -> Sum/1
  PosOut/1 -> Sum/2
  VelRef/1 -> Sum1/1
  VelOut/1 -> Sum1/2
  Sum1/1 -> Gain/1
  Sum/1 -> Gain1/1
  Gain1/1 -> Sum2/1
  Gain/1 -> Sum2/2
  Sum2/1 -> Force/1

== system Master_Slave_Model/SLAVE_SIDE /Velocity Approx + LPF  ==
  Pos : Inport
  Clock : simulink_extras/Flip Flops/Clock  period=Ts*2
  Clock1 : simulink_extras/Flip Flops/Clock  period=Ts*2
  Constant : Constant  Value=Ts
  Constant1 : Constant  Value=beta
  "Euler Approximation " : MATLAB Function  TreatAsAtomicUnit=on
  Sample and Hold : dspsigops/Sample and Hold  trig=Rising edge  initCond=0  latchinput=on
  Sample and Hold1 : dspsigops/Sample and Hold  trig=Rising edge  initCond=0  latchinput=on
  "Vel_H_LPF " : Outport
  wires:
  Pos/1 -> Sample and Hold/1, "Euler Approximation "/3(pos)
  Constant/1 -> "Euler Approximation "/2(Ts)
  Sample and Hold/1 -> "Euler Approximation "/4(posPrev)
  Clock/1 -> Sample and Hold/Trigger
  Sample and Hold1/1 -> "Euler Approximation "/5(filteredPrev)
  "Euler Approximation "/1(filtered) -> "Vel_H_LPF "/1, Sample and Hold1/1
  Clock1/1 -> Sample and Hold1/Trigger
  Constant1/1 -> "Euler Approximation "/1(beta)

== system Master_Slave_Model/SLAVE_SIDE /Zh_hat - Impedance Controller ==
  Error_Vel_MF : Inport
  Operator Stifness : Inport  Port=2
  Discrete-Time Integrator1 : DiscreteIntegrator  SampleTime=Ts  ICPrevOutput=DiscIntNeverNeededParam  ICPrevScaledInput=DiscIntNeverNeededParam
  Gain : Gain  Gain=Bh
  Gain1 : Gain  Gain=Kh
  Integrator : Integrator
  Product : Product
  Sum : Sum
  "Force_Zh_hat " : Outport
  wires:
  Error_Vel_MF/1 -> Integrator/1, Gain/1
  Gain/1 -> Sum/1
  Gain1/1 -> Sum/2
  Sum/1 -> "Force_Zh_hat "/1
  Operator Stifness/1 -> ?
  Integrator/1 -> Gain1/1

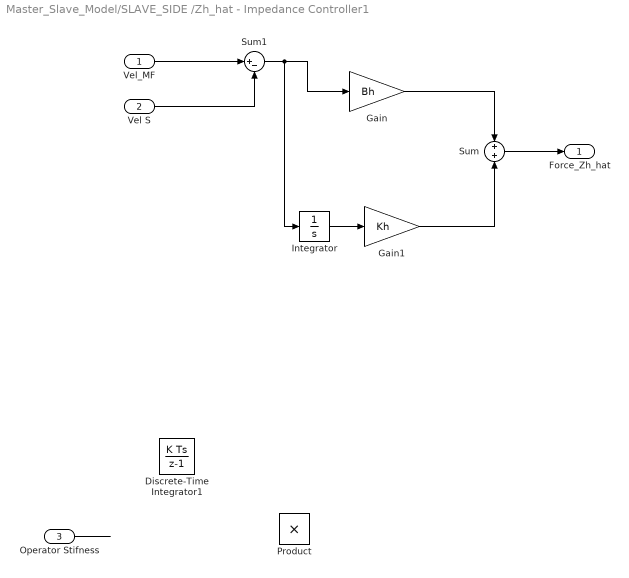
== system Master_Slave_Model/SLAVE_SIDE /Zh_hat - Impedance Controller1 ==
  Vel_MF : Inport
  Vel S : Inport  Port=2
  Operator Stifness : Inport  Port=3
  Discrete-Time Integrator1 : DiscreteIntegrator  SampleTime=Ts  ICPrevOutput=DiscIntNeverNeededParam  ICPrevScaledInput=DiscIntNeverNeededParam
  Gain : Gain  Gain=Bh
  Gain1 : Gain  Gain=Kh
  Integrator : Integrator
  Product : Product
  Sum : Sum
  Sum1 : Sum  Inputs=|+-
  "Force_Zh_hat " : Outport
  wires:
  Integrator/1 -> Gain1/1
  Operator Stifness/1 -> ?
  Sum/1 -> "Force_Zh_hat "/1
  Gain1/1 -> Sum/2
  Gain/1 -> Sum/1
  Vel_MF/1 -> Sum1/1
  Sum1/1 -> Integrator/1, Gain/1
  Vel S/1 -> Sum1/2

== system Master_Slave_Model/POPC - Master Side/PO Input - Slave to Master (Cause)/PASSIVE OBSERVER S2M E Right INPUT ==
  Env_Force : Inport
  "Vel_M " : Inport  Port=2
  Clock : simulink_extras/Flip Flops/Clock  period=Ts*2
  Product : Product
  Sample and Hold : dspsigops/Sample and Hold  trig=Rising edge  initCond=0  latchinput=on
  Sum : Sum
  E-Rin : Outport
  wires:
  Env_Force/1 -> Product/1
  "Vel_M "/1 -> Product/2
  Product/1 -> Sum/2
  Sum/1 -> Sample and Hold/1, E-Rin/1
  Sample and Hold/1 -> Sum/1
  Clock/1 -> Sample and Hold/Trigger

== system Master_Slave_Model/POPC - Master Side/PO Output - Master to Slave (Effect)/PASSIVE OBSERVER M2S E Left OUTPUT ==
  Velocity Master : Inport
  Force Env Delayed : Inport  Port=2
  Clock : simulink_extras/Flip Flops/Clock  period=Ts*2
  Product : Product
  Sample and Hold : dspsigops/Sample and Hold  trig=Rising edge  initCond=0  latchinput=on
  Sum : Sum
  E-Lout : Outport
  wires:
  Velocity Master/1 -> Product/1
  Force Env Delayed/1 -> Product/2
  Product/1 -> Sum/2
  Sample and Hold/1 -> Sum/1
  Sum/1 -> Sample and Hold/1, E-Lout/1
  Clock/1 -> Sample and Hold/Trigger

== matlab function Master_Slave_Model/POPC - Master Side/PC - Master side/PASSIVE CONTROLLER PCm ==
  data: E_POm input; E_PCm output; dt input; v_m input; E_PCm_prev input; alpha_m output
function [E_PCm, alpha_m]= PC_m(E_POm, dt, v_m, E_PCm_prev)

if (E_POm < 0 && v_m ~= 0)
    alpha_m = (-E_POm)/dt*v_m^2;
else
    alpha_m = 0;
end

E_PCm = E_PCm_prev + (alpha_m*v_m^2)*dt;

== matlab function Master_Slave_Model/SLAVE_SIDE /Euler Approximation Vel MH1/Euler Approximation  ==
  data: beta input; Ts input; filtered output; pos input; posPrev input; filteredPrev input
function filtered = EulApprox(beta, Ts, pos, posPrev, filteredPrev)

eul= (pos - posPrev)/Ts;
filtered = beta*eul + (1-beta)*filteredPrev;

== matlab function Master_Slave_Model/MASTER SIDE/Velocity Approx + LPF 3/Euler Approximation  ==
  data: beta input; Ts input; filtered output; pos input; posPrev input; filteredPrev input
function filtered = EulApprox(beta, Ts, pos, posPrev, filteredPrev)

eul= (pos - posPrev)/Ts;
filtered = beta*eul + (1-beta)*filteredPrev;

== matlab function Master_Slave_Model/SLAVE_SIDE /Environment /Environment Behaviour ==
  data: x_s input; Fe output; dot_x_s input; qe input; Be input; Ke input
function Fe = Env(x_s, dot_x_s, qe, Be, Ke)
    
    if(x_s > qe)
        Fe = Ke*(x_s - qe) + Be*dot_x_s;
    else
        Fe = 0;
    end

== matlab function Master_Slave_Model/Operator Stiffness/Operator Stiffness  ==
  data: KhMax input; Kh input; Kh_func output; t input; stopTime input
function Kh_func = stiffness(KhMax, Kh, t, stopTime)
%Solving cubic polynomial function to model the operator stiffness
%(f'(begin) + f'(end) - 2*f(begin))(x/k)^3 + (3*f(end) - 2*f'(begin) - f'(end))(x/k)^2 + f'(begin)x/k + f(begin)

    begin = 0.5;

    endTime = stopTime-0.5;

    df_begin = 0;
    df_end = 0;
    f_end = KhMax - Kh;

    if t < begin
    Kh_func = Kh;
    else
    Kh_func = (df_begin + df_end - 2*f_end)*((t-begin)/endTime)^3 + (3*f_end - 2*df_begin - df_end)*((t-begin)/endTime)^2 + (df_begin)*((t-begin)/endTime) + Kh;
    end
end

== matlab function Master_Slave_Model/POPC - Slave Side/PC Slave/PASSIVE CONTROLLER PCs ==
  data: E_PCs_prev input; E_POs input; E_PCs output; dt input; v_s input; alpha_s output
function [E_PCs, alpha_s]= PC_s(E_PCs_prev, E_POs, dt, v_s)

if (E_POs < 0 && v_s ~= 0)
    alpha_s = (-E_POs)/dt*v_s^2;
else
    alpha_s = 0;
end

E_PCs = E_PCs_prev + (alpha_s*v_s^2)*dt;

== matlab function Master_Slave_Model/SLAVE_SIDE /Velocity Approx + LPF /Euler Approximation  ==
  data: beta input; Ts input; filtered output; pos input; posPrev input; filteredPrev input
function filtered = EulApprox(beta, Ts, pos, posPrev, filteredPrev)

eul= (pos - posPrev)/Ts;
filtered = beta*eul + (1-beta)*filteredPrev;

== matlab function Master_Slave_Model/Euler Approximation Vel M1/Euler Approximation  ==
  data: beta input; Ts input; filtered output; pos input; posPrev input; filteredPrev input
function filtered = EulApprox(beta, Ts, pos, posPrev, filteredPrev)

eul= (pos - posPrev)/Ts;
filtered = beta*eul + (1-beta)*filteredPrev;

== matlab function Master_Slave_Model/MASTER SIDE/Velocity Approx + LPF 1/Euler Approximation  ==
  data: beta input; Ts input; filtered output; pos input; posPrev input; filteredPrev input
function filtered = EulApprox(beta, Ts, pos, posPrev, filteredPrev)

eul= (pos - posPrev)/Ts;
filtered = beta*eul + (1-beta)*filteredPrev;

== matlab function Master_Slave_Model/MASTER SIDE/Velocity Approx + LPF 2/Euler Approximation  ==
  data: beta input; Ts input; filtered output; pos input; posPrev input; filteredPrev input
function filtered = EulApprox(beta, Ts, pos, posPrev, filteredPrev)

eul= (pos - posPrev)/Ts;
filtered = beta*eul + (1-beta)*filteredPrev;

== matlab function Master_Slave_Model/MASTER SIDE/Velocity Approx + LPF /Euler Approximation  ==
  data: beta input; Ts input; filtered output; pos input; posPrev input; filteredPrev input
function filtered = EulApprox(beta, Ts, pos, posPrev, filteredPrev)

eul= (pos - posPrev)/Ts;
filtered = beta*eul + (1-beta)*filteredPrev;
